simulink model "SecRwLtStHdrstFwdBkwdHolderChk"  (R2018b)
settings: Solver=FixedStepDiscrete  StartTime=0.0  StopTime=10.0  FixedStep=0.01  RelTol=1e-3
libraries: simulink x1
settings Model: Creator=sn2xws  LastModifiedBy=sn2xws
settings Model: ModifiedHistory=|
  | 2023/11/7
  | BUG 555794 童锁停止模式21-26
settings DataIOCC: SaveFormat=StructureWithTime
settings OptimizationCC: DefaultParameterBehavior=Inlined  EnhancedBackFolding=on  PassReuseOutputArgsAs=Individual arguments  ZeroExternalMemoryAtStartup=off  ZeroInternalMemoryAtStartup=off  OptimizeBlockOrder=speed  DifferentSizesBufferReuse=on  OptimizationCustomize=off
settings DebuggingCC: ParameterTunabilityLossMsg=error
settings ModelReferenceCC: ModelReferenceNumInstancesAllowed=Single
settings SFSimCC: MATLABDynamicMemAlloc=off
settings RTWCC: SystemTargetFile=autosar.tlc  GenCodeOnly=on  TemplateMakefile=ert_default_tmf  Description=AUTOSAR  GenerateReport=on  IncludeHyperlinkInReport=on  LaunchReport=on  GenerateTraceInfo=on  GenerateTraceReport=on  GenerateTraceReportSl=on  GenerateTraceReportSf=on  GenerateTraceReportEml=on
settings CodeAppCC: ForceParamTrailComments=on  IgnoreCustomStorageClasses=off  OperatorAnnotations=on  SimulinkDataObjDesc=on  SFDataObjDesc=on  InsertBlockDesc=on
settings STFCustomTargetCC: TargetLangStandard=C99 (ISO)  MultiwordLength=256  ParMdlRefBuildCompliant=on  CompOptLevelCompliant=on  IncludeMdlTerminateFcn=off  CombineOutputUpdateFcns=on  SuppressErrorStatus=on  ERTCustomFileBanners=on  SupportNonFinite=off  SupportComplex=off  SupportContinuousTime=off  SupportNonInlinedSFcns=off  RemoveResetFunc=on  MATLABClassNameForMDSCustomization=Simulink.SoftwareTarget.ERTCustomization  AutosarCompliant=on  UseToolchainInfoCompliant=on  LookupTableObjectStructAxisOrder=2,1,3,4,...  LUTObjectStructOrderEvenSpacing=Size,Table,Breakpoints  SystemTargetFile=autosar.tlc
settings ERTTargetCC: TargetLangStandard=C99 (ISO)  ConcurrentExecutionCompliant=off  IncludeMdlTerminateFcn=off  SuppressErrorStatus=on  SupportNonFinite=off  SupportComplex=off  ModelStepFunctionPrototypeControlCompliant=off  CPPClassGenCompliant=off  AutosarCompliant=on  LookupTableObjectStructAxisOrder=2,1,3,4,...  LUTObjectStructOrderEvenSpacing=Size,Table,Breakpoints  InlinedParameterPlacement=NonHierarchical  ERTCustomFileTemplate=example_file_process.tlc  ERTFilePackagingFormat=Compact

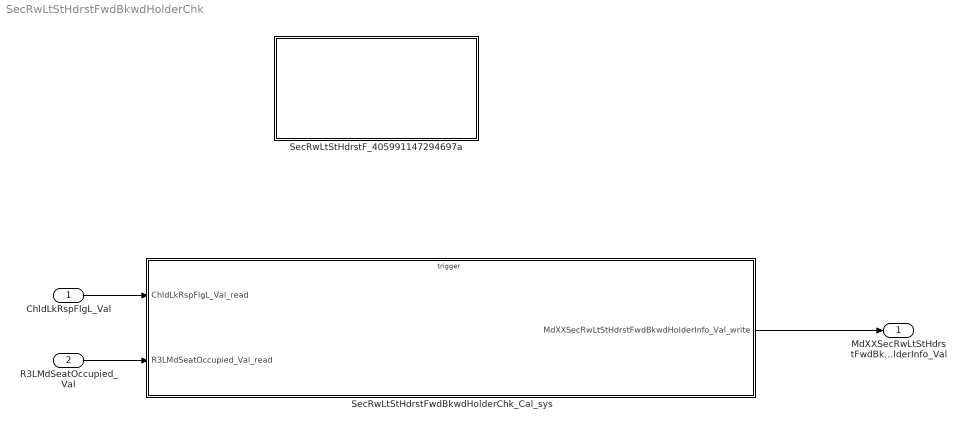
== system SecRwLtStHdrstFwdBkwdHolderChk ==
  ChldLkRspFlgL_Val : Inport  OutDataTypeStr=boolean  PortDimensions=1
  R3LMdSeatOccupied_Val : Inport  Port=2  OutDataTypeStr=boolean  PortDimensions=1
  SecRwLtStHdrstF_405991147294697a : Subsystem
  SecRwLtStHdrstFwdBkwdHolderChk_Cal_sys : Subsystem
  MdXXSecRwLtStHdrstFwdBkwdHolderInfo_Val : Outport  OutDataTypeStr=uint32  PortDimensions=1
  wires:
  ChldLkRspFlgL_Val/1 -> SecRwLtStHdrstFwdBkwdHolderChk_Cal_sys/1(ChldLkRspFlgL_Val_read)
  R3LMdSeatOccupied_Val/1 -> SecRwLtStHdrstFwdBkwdHolderChk_Cal_sys/2(R3LMdSeatOccupied_Val_read)
  SecRwLtStHdrstFwdBkwdHolderChk_Cal_sys/1(MdXXSecRwLtStHdrstFwdBkwdHolderInfo_Val_write) -> MdXXSecRwLtStHdrstFwdBkwdHolderInfo_Val/1

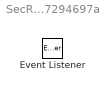
== system SecRwLtStHdrstFwdBkwdHolderChk/SecRwLtStHdrstF_405991147294697a ==
  Event Listener : EventListener  EventName=reset

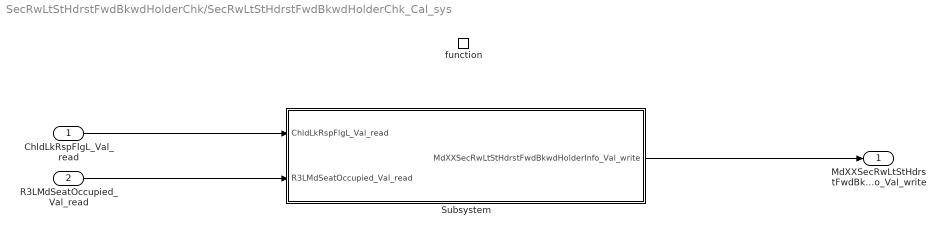
== system SecRwLtStHdrstFwdBkwdHolderChk/SecRwLtStHdrstFwdBkwdHolderChk_Cal_sys ==
  ChldLkRspFlgL_Val_read : Inport
  R3LMdSeatOccupied_Val_read : Inport  Port=2
  function : TriggerPort  TriggerType=function-call  IsSimulinkFunction=on  FunctionName=SecRwLtStHdrstFwdBkwdHolderChk_Cal  VariantControl=(inherit)
  Subsystem : Subsystem
  MdXXSecRwLtStHdrstFwdBkwdHolderInfo_Val_write : Outport
      settings: EnsureOutportIsVirtual=on
  wires:
  Subsystem/1(MdXXSecRwLtStHdrstFwdBkwdHolderInfo_Val_write) -> MdXXSecRwLtStHdrstFwdBkwdHolderInfo_Val_write/1
  ChldLkRspFlgL_Val_read/1 -> Subsystem/1(ChldLkRspFlgL_Val_read)
  R3LMdSeatOccupied_Val_read/1 -> Subsystem/2(R3LMdSeatOccupied_Val_read)

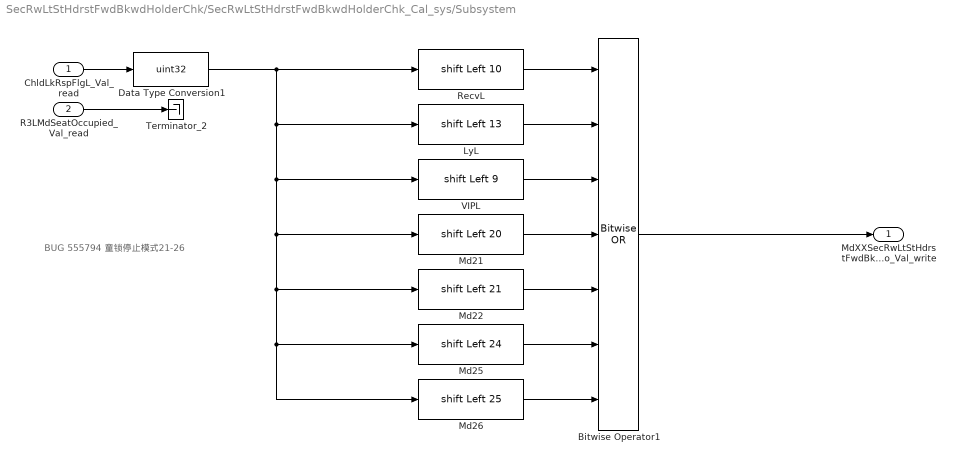
== system SecRwLtStHdrstFwdBkwdHolderChk/SecRwLtStHdrstFwdBkwdHolderChk_Cal_sys/Subsystem ==
  note: BUG 555794 童锁停止模式21-26
  ChldLkRspFlgL_Val_read : Inport
  R3LMdSeatOccupied_Val_read : Inport  Port=2
  Bitwise Operator1 : simulink/Logic and Bit Operations/Bitwise Operator  logicop=OR  UseBitMask=off  NumInputPorts=7  BitMask=bin2dec('11011001')  BitMaskRealWorld=Stored Integer
  Data Type Conversion1 : DataTypeConversion  OutDataTypeStr=uint32
  LyL : ArithShift  BitShiftNumber=13  BitShiftDirection=Left
  Md21 : ArithShift  BitShiftNumber=20  BitShiftDirection=Left
  Md22 : ArithShift  BitShiftNumber=21  BitShiftDirection=Left
  Md25 : ArithShift  BitShiftNumber=24  BitShiftDirection=Left
  Md26 : ArithShift  BitShiftNumber=25  BitShiftDirection=Left
  RecvL : ArithShift  BitShiftNumber=10  BitShiftDirection=Left
  Terminator_2 : Terminator
  VIPL : ArithShift  BitShiftNumber=9  BitShiftDirection=Left
  MdXXSecRwLtStHdrstFwdBkwdHolderInfo_Val_write : Outport
      settings: EnsureOutportIsVirtual=on
  wires:
  R3LMdSeatOccupied_Val_read/1 -> Terminator_2/1
  Bitwise Operator1/1 -> MdXXSecRwLtStHdrstFwdBkwdHolderInfo_Val_write/1
  ChldLkRspFlgL_Val_read/1 -> Data Type Conversion1/1
  Data Type Conversion1/1 -> RecvL/1, Md26/1, Md25/1, Md22/1, Md21/1, VIPL/1, LyL/1
  VIPL/1 -> Bitwise Operator1/3
  LyL/1 -> Bitwise Operator1/2
  RecvL/1 -> Bitwise Operator1/1
  Md21/1 -> Bitwise Operator1/4
  Md22/1 -> Bitwise Operator1/5
  Md25/1 -> Bitwise Operator1/6
  Md26/1 -> Bitwise Operator1/7
